simulink model "sensorFusionWithControlBackup"  (R2024a)
settings: Solver=FixedStepAuto  StartTime=0.0  StopTime=inf  FixedStep=controlRate  RelTol=1e-3  EnableMultiTasking=on
InitFcn:
  | motorParamsDD = Simulink.data.dictionary.open('motorParametersData.sldd');
  | robotParamsDD = Simulink.data.dictionary.open('robotModelData.sldd');
  | controlParamsDD = Simulink.data.dictionary.open('controlVariablesData.sldd');
  | modelParamsDD = Simulink.data.dictionary.open('modelConfigData.sldd');
  | sectMotor = getSection(motorParamsDD,'Design Data');
  | sectRobot = getSection(robotParamsDD,'Design Data');
  | sectControl = getSection(controlParamsDD,'Design Data');
  | sectModel = getSection(modelParamsDD,'Design Data');
  | 
  | %% Physical Parameters
  | M = getValue(getEntry(sectRobot,'massOfCart'));    % mass of cart
  | m = getValue(getEntry(sectRobot,'massOfPendulum'));    % mass of pendulum
  | L = getValue(getEntry(sectRobot,'lengthToPendulumCenterOfMass'));    % length to pendulum center of mass
  | g = 9.81;   % gravity
  | I = getValue(getEntry(sectRobot,'inertiaOfPendulum'));  % inertia of pendulum
  | r = getValue(getEntry(sectRobot,'wheelRadius'));   % 5 cm wheel radius
  | 
  | % Servo motor state: i, omega
  | Rm = getValue(getEntry(sectMotor,'armatureResistance')); % motor resistance
  | Lm = getValue(getEntry(sectMotor,'armatureInductance')); % motor coil inductance
  | Km = getValue(getEntry(sectMotor,'motorTorqueConstantKm')); % motor torque constant
  | Kb = getValue(getEntry(sectMotor,'backEMFConstantKb')); % motor electrical consant
  | Kf = getValue(getEntry(sectMotor,'viscousFriction')); % viscous friction
  | J = getValue(getEntry(sectMotor,'motorInertia'));  % inertia of rotor
  | 
  | 
  | Q_lqr_temp = getValue(getEntry(sectControl,'Q_lqr'));
  | R_lqr_temp = getValue(getEntry(sectControl,'R_lqr'));
  | Q_aug_lqr_temp = getValue(getEntry(sectControl,'Q_aug_lqr'));
  | R_aug_lqr_temp = getValue(getEntry(sectControl,'R_aug_lqr'));
  | 
  | % States are x, dx/dt, phi, dphi/dt
  | % Outputs are x position and tilt angle
  | 
  | % Linearized state-space model of inverted pendulum
  | I_tot = m*L^2+I;
  | p = m^2*L^2 - I_tot*(M+m);
  | A_pend = [0 1 0 0;
  |           0 0 (m^2 * g * L^2)/p 0;
  |           0 0 0 1;
  |           0 0 -(M+m)/(m*L)*m^2*L^2*g/p 0];
  | 
  | B_pend = [0; -I_tot/p; 0; 1/(m*L)*(1+(M+m)*I_tot/p)];
  | 
  | C_pend = [1 0 0 0;
  |           0 0 1 0];
  | D_pend = zeros(2,1);
  | 
  | % Discretize System - for the augmented system
  | dt = getValue(getEntry(sectModel,'stateEstRate'));
  | sysd = c2d(ss(A_pend, B_pend, C_pend, D_pend), dt);
  | Ad_pend = single(sysd.A);
  | Bd_pend = single(sysd.B);
  | Cd_pend = single(sysd.C);
  | Dd_pend = single(sysd.D);
  | 
  | % LQR Controller - for the augmented system
  | % Q_lqr = diag([1/0.02^2 1/0.1^2 1/(10*pi/180)^2 1/0.1^2]);
  | % R_lqr = 1;
  | [K_lqr, ~, ~] = dlqr(Ad_pend, Bd_pend, Q_lqr_temp, R_lqr_temp);
  | K_lqr = single(K_lqr);
  | 
  | % State-space model: output is torque = Km * i
  | A_motor = [-Rm/L,   -Kb/Lm;
  |             Km/J, -Kf/J];
  | B_motor = [1/Lm;
  |            0];
  | C_motor = [Km*(1/r), 0];  % Output is torque = Km * i
  | D_motor = 0;
  | 
  | % Augment System: Force = torque / r
  | % States are x, dx/dt, phi, dphi/dt, i, w
  | % Outputs are x position and tilt angle
  | 
  | A_aug = [A_pend, B_pend*C_motor;
  |          zeros(2,4), A_motor];
  | 
  | B_aug = [B_pend*D_motor; B_motor];
  | 
  | C_aug = [C_pend, D_pend*C_motor];
  | n_aug = size(A_aug,1);
  | 
  | 
  | % Discretize System - for the augmented system
  | sysd = c2d(ss(A_aug, B_aug, C_aug, 0), dt);
  | Ad_aug = single(sysd.A);
  | Bd_aug = single(sysd.B);
  | Cd_aug = single(sysd.C);
  | 
  | clear J Kt M m l g I r Q_lqr_temp R_lqr_temp dt
  | clear Rm Lm Km Kb Kf J
  | clear motorParamsDD robotParamsDD controlParamsDD modelParamsDD sectMotor sectRobot sectControl sectModel
  | 
  | 
  | % LQR Controller - for the augmented system
  | % Q_aug = diag([1/0.02^2 1/0.1^2 1/(10*pi/180)^2 1/0.1^2 1 1]);
  | % R_aug_lqr = 1;
  | [K_aug_lqr, ~, ~] = dlqr(Ad_aug, Bd_aug, Q_aug_lqr_temp, R_aug_lqr_temp);
  | K_aug_lqr = single(K_aug_lqr);
  | % K_aug_lqr = single([0.0 0.0 -39.4009209 -5.59002447 0.293991983 -0.0311870389])
  | 
  | clear Q_aug_lqr_temp R_aug_lqr_temp
  | 
  | % % Kalman Filter - for the augmented system
  | % Q_kf = diag([0.02 0.02 0.02 0.02]);   % Slightly higher process noise
  | % Q_kf_aug = diag([0.02 0.02 0.02 0.02 0.02 0.02]);   % Slightly higher process noise
  | % R_kf = 0.01*diag([0.001 0.001]);                 % Lower measurement noise (trust sensors more)
undefined symbols (not defined in the file): accelToUnit, angleEstRate, controlRate, CPR, D_min, DiscIntNeverNeededParam, Dmin, gyroToUnit, MaxMotorVoltage, Q_ang_kf, R_ang_kf, stateEstRate, wheelBase, wheelRadius
libraries: stm32f4xxblockslib x13, dspstat3 x6, stm32blockslib x2, stm32f7xxblockslib x2, slpidlib x1
settings Model: DataDictionary=globalData.sldd  VariantConfigurationObject=RobotVariantConfig  STM32="{\"DigitalPortWrite\":[{\"ID\":\"sensorFusionWithControlBackup:191\"},{\"ID\":\"sensorFusionWithControlBackup:197\"},{\"ID\":\"sensorFusionWithControlBackup:199\"},{\"ID\":\"sensorFusionWithControlBackup:201\"},{\"ID\":\"sensorFusionWithControlBackup:203\"},{\"ID\":\"sensorFusionWithControlBackup:667\"},{\"ID\":\"sensorFusionWithControlBackup:668\"},{\"ID\":\"sensorFusionWithControlBackup:669\"},{\"ID\":\"sensorFusionWithControlBackup:670\"},{\"ID\":\"sensorFusionWithControlBackup:778\"},{\"ID\":\"sensorFusionWithControlBackup:779\"},{\"ID\":\"sensorFusionWithControlBackup:780\"},{\"ID\":\"sensorFusionWithControlBackup:781\"}],\"PWMOutput\":[{\"ID\":\"sensorFusionWithControlBackup:205\"},{\"ID\":\"sensorFusionWithControlBackup:189\"}],\"EncoderBlock\":[{\"ID\":\"sensorFusionWithControlBackup:932\"},{\"ID\":\"sensorFusionWithControlBackup:935\"}],\"I2CControllerRead\":[{\"ID\":\"sensorFusionWithControlBackup:63:801\"},{\"ID\":\"sensorFusionWithControlBackup:63:802\"},{\"ID\":\"sensorFusionWithControlBackup:63:803\"},{\"ID\":\"sensorFusionWithControlBackup:63:804\"},{\"ID\":\"sensorFusionWithControlBackup:63:799\"},{\"ID\":\"sensorFusionWithControlBackup:63:800\"},{\"ID\":\"sensorFusionWithControlBackup:63:813\"},{\"ID\":\"sensorFusionWithControlBackup:63:814\"},{\"ID\":\"sensorFusionWithControlBackup:78:799\"},{\"ID\":\"sensorFusionWithControlBackup:78:800\"},{\"ID\":\"sensorFusionWithControlBackup:78:801\"},{\"ID\":\"sensorFusionWithControlBackup:78:802\"},{\"ID\":\"sensorFusionWithControlBackup:78:803\"},{\"ID\":\"sensorFusionWithControlBackup:78:804\"},{\"ID\":\"sensorFusionWithControlBackup:78:812\"},{\"ID\":\"sensorFusionWithControlBackup:78:813\"},{\"ID\":\"sensorFusionWithControlBackup:78:814\"}],\"I2CControllerWrite\":[{\"ID\":\"sensorFusionWithControlBackup:63:815\"},{\"ID\":\"sensorFusionWithControlBackup:63:816\"},{\"ID\":\"sensorFusionWithControlBackup:78:815\"},{\"ID\":\"sensorFusionWithControlBackup:78:816\"},{\"ID\":\"sensorFusionWithControlBackup:78:817\"}]}"  SimulationMode=external  Creator=Peter  LastModifiedBy=Peter
settings OptimizationCC: EnhancedBackFolding=on  PassReuseOutputArgsAs=Individual arguments  ZeroExternalMemoryAtStartup=off  ZeroInternalMemoryAtStartup=off  MaxStackSize=64  OptimizeBlockOrder=speed  DifferentSizesBufferReuse=on  OptimizationCustomize=off  EfficientTunableParamExpr=on
settings DebuggingCC: ParameterTunabilityLossMsg=error
settings HardwareCC: ProdBitPerPointer=32  ProdBitPerSizeT=32  ProdBitPerPtrDiffT=32  ProdLargestAtomicInteger=Long  ProdLargestAtomicFloat=Double  ProdWordSize=32  ProdLongLongMode=on  ProdHWDeviceType=ARM Compatible->ARM Cortex-M
settings SFSimCC: MATLABDynamicMemAlloc=off
settings RTWCC: Description=Embedded Coder  SystemTargetFile=ert.tlc  HardwareBoard=STM32F7xx Based (Single precision FPU)  TemplateMakefile=ert_default_tmf  Toolchain=GNU Tools for ARM Embedded Processors
settings CodeAppCC: ForceParamTrailComments=on  IgnoreCustomStorageClasses=off  OperatorAnnotations=on  SimulinkDataObjDesc=on  SFDataObjDesc=on  InsertBlockDesc=on
settings ERTTargetCC: TargetLangStandard=C99 (ISO)  CodeReplacementLibrary=ARM Cortex-M  ExtMode=on  ExtModeTransport=3  ExtModeStaticAlloc=on  ExtModeStaticAllocSize=2048  ExtModeMexFile=ext_xcp  ExtModeMexArgs=1 'COM11' 115200  ExtModeIntrfLevel=Level2 - Open

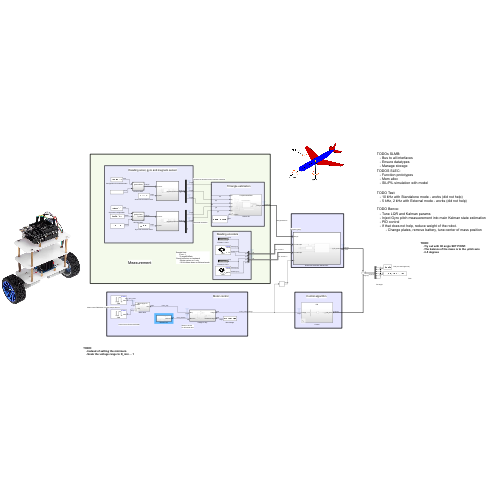
[thumbnail: Simulink's stored preview of the top-level diagram]
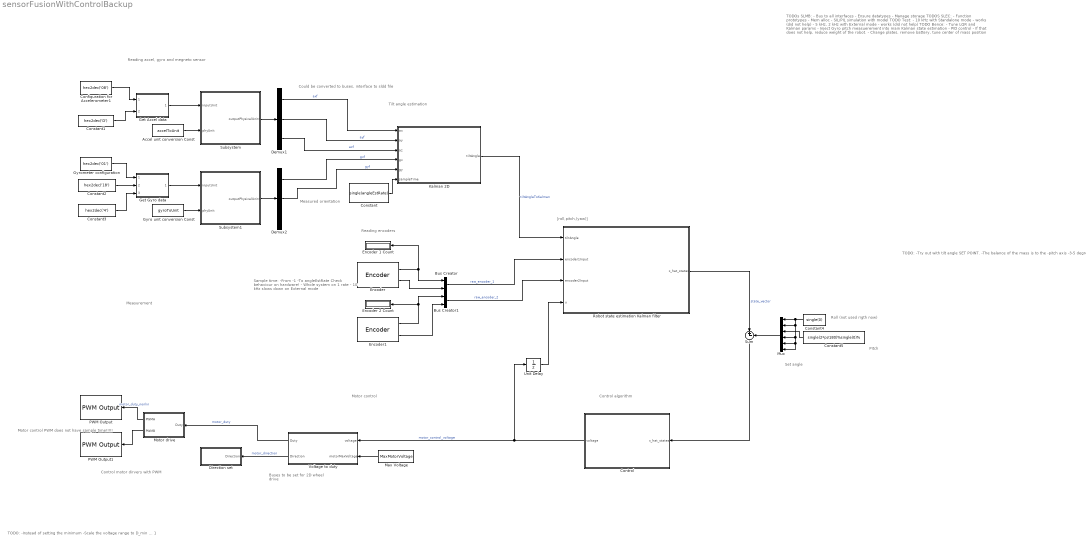
== system sensorFusionWithControlBackup ==
  note: Pitch
  note: Roll (not used rigth now)
  note: Set angle
  note: TODO:
      | -Try out with tilt angle SET POINT.
      | -The balance of the mass is to the -pitch axis
      | -3-5 degrees
  note: Measured orientation
  note: TODOs SLMB:
      | - Bus to all interfaces
      | - Ensure datatypes
      | - Manage storage
      | TODOS SLEC:
      | - Function prototypes
      | - Mem alloc
      | - SIL/PIL simulation with model
      |
      | TODO Test:
      | - 10 kHz with Standalone mode - works (did not help)
      | - 5 kHz, 2 kHz with External mode - works (did not help)
      |
      | TODO Bence:
      | - Tune LQR and Kalman params
      | - Inject Gyro pitch measuerement into main Kalman state estimation
      | - PID control
      | - If that does not help, reduce weight of the robot.
      | - Change plates, remove battery, tune center of mass position
  note: Motor control PWM does not have sample time!!!!!
  note: Sample time:
      | -From -1
      | -To angleEstRate
      | Check behaviour on hardware!
      | - Whole system on 1 rate
      | - 10 kHz slows down on External mode
  note: Measurement
  note: Motor control
  note: Tilt angle estimation
  note: Buses to be set
      | for 2D wheel drive
  note: Control motor dirvers with PWM
  note: Could be converted to buses, interface to sldd file
  note: Reading accel, gyro and megneto sensor
  note: Control algorithm
  note: TODO:
      | -Instead of setting the minimum
      | -Scale the voltage range to D_min ... 1
  note: [roll,pitch,(yaw)]
  note: Reading encoders
  Accel unit conversion Const : Constant  Value=accelToUnit  OutDataTypeStr=single
  Bus Creator : BusCreator  Inputs=2
  Bus Creator1 : BusCreator  Inputs=2
  Configuration for Accelerometer1 : Constant  Value=hex2dec('08')  OutDataTypeStr=uint8
  Constant : Constant  Value=single(angleEstRate)  OutDataTypeStr=single
  Constant1 : Constant  Value=hex2dec('D')  OutDataTypeStr=uint8
  Constant2 : Constant  Value=hex2dec('18')
  Constant3 : Constant  Value=hex2dec('4')
  Constant4 : Constant  Value=single(0)
  Constant5 : Constant  Value=single(2*pi/180)%single(0)%
  Control : Subsystem  Variant=on  VariantControl=Subsystem2  VariantActivationTime=inherit from Simulink.VariantControl
  Demux1 : Demux  Outputs=3
  Demux2 : Demux  Outputs=3
  Direction set : Subsystem  TreatAsAtomicUnit=on  SystemSampleTime=controlRate
  Encoder : stm32blockslib/Encoder  TimerModule=TIM1  EnableResetInput=off  OutputDirection=on  SampleTime=angleEstRate
      settings: LibrarySourceBlock=stm32f7xxblockslib/Encoder
  Encoder 1 Count : Display
      settings: Format=hex (Stored Integer)
  Encoder 2 Count : Display
      settings: Format=hex (Stored Integer)
  Encoder1 : stm32blockslib/Encoder  TimerModule=TIM3  EnableResetInput=off  OutputDirection=on  SampleTime=angleEstRate
      settings: LibrarySourceBlock=stm32f7xxblockslib/Encoder
  Get Accel data : Subsystem  TreatAsAtomicUnit=on  SystemSampleTime=angleEstRate  ReferencedSubsystem=getAccelData
  Get Gyro data : Subsystem  TreatAsAtomicUnit=on  SystemSampleTime=angleEstRate  ReferencedSubsystem=getGyroData
  Gyro unit conversion Const : Constant  Value=gyroToUnit  OutDataTypeStr=single
  Gyrometer configuration : Constant  Value=hex2dec('01')  OutDataTypeStr=uint8
  Kalman 2D : Subsystem  Variant=on  VariantControl=Kalman 2D  VariantActivationTime=inherit from Simulink.VariantControl
  Max Voltage : Constant  Value=MaxMotorVoltage  OutDataTypeStr=single
  Motor drive : Subsystem  Variant=on  VariantControl=Motor drive  VariantActivationTime=inherit from Simulink.VariantControl
  Mux : Mux  Inputs=6
  PWM Output : stm32f7xxblockslib/PWM Output  TimerModule=TIM8  DutycycleUnits=Percentage  EnableChannel1=off  EnableChannel2=off  EnableChannel3=on  EnableChannel4=off  EnableChannel5=off  EnableChannel6=off  EnableCounterInput=off  EnableMainOutputInput=off  EnableFrequencyInput=off  SetRCAfterCE=off  OutputDirection=off  OutputMainOutputEnableStatus=off  SampleTime=0.1  EnableSimPort=off  EnableUpdateEvent=off  EnableCaptureCompare1Event=off  EnableCaptureCompare2Event=off  EnableCaptureCompare3Event=off  EnableCaptureCompare4Event=off  EnableTriggerEvent=off  EnableBreakEvent=off  EnableBreakEvent2=off  ProcessorFamily=STM32F7  hoistedMaskSrc=ECSoC/ECSimCodegen/PWM Output
  PWM Output1 : stm32f7xxblockslib/PWM Output  TimerModule=TIM8  DutycycleUnits=Percentage  EnableChannel1=off  EnableChannel2=off  EnableChannel3=off  EnableChannel4=on  EnableChannel5=off  EnableChannel6=off  EnableCounterInput=off  EnableMainOutputInput=off  EnableFrequencyInput=off  SetRCAfterCE=off  OutputDirection=off  OutputMainOutputEnableStatus=off  SampleTime=0.1  EnableSimPort=off  EnableUpdateEvent=off  EnableCaptureCompare1Event=off  EnableCaptureCompare2Event=off  EnableCaptureCompare3Event=off  EnableCaptureCompare4Event=off  EnableTriggerEvent=off  EnableBreakEvent=off  EnableBreakEvent2=off  ProcessorFamily=STM32F7  hoistedMaskSrc=ECSoC/ECSimCodegen/PWM Output
  Robot state estimation Kalman filter : Subsystem  TreatAsAtomicUnit=on  SystemSampleTime=stateEstRate
  Subsystem : Subsystem  TreatAsAtomicUnit=on  SystemSampleTime=angleEstRate
  Subsystem1 : Subsystem  TreatAsAtomicUnit=on  SystemSampleTime=angleEstRate
  Sum : Sum  Inputs=|+-
  Unit Delay : UnitDelay  SampleTime=controlRate  HasFrameUpgradeWarning=on
  Voltage to duty : Subsystem  TreatAsAtomicUnit=on  SystemSampleTime=controlRate
  wires:
  Motor drive/1(PWMA) -> PWM Output/1  "motor_duty_nonlin"
  Motor drive/2(PWMB) -> PWM Output1/1
  Voltage to duty/1(Duty) -> Motor drive/1(Duty)  "motor_duty"
  Voltage to duty/2(Direction) -> Direction set/1(Direction)  "motor_direction"
  Max Voltage/1 -> Voltage to duty/2(motorMaxVoltage)
  Gyro unit conversion Const/1 -> Subsystem1/2(phyUnit)
  Subsystem1/1(outputPhysicalUnits) -> Demux2/1
  Gyrometer configuration/1 -> Get Gyro data/1
  Get Gyro data/1 -> Subsystem1/1(inputUnit)
  Demux1/1 -> Kalman 2D/1(ax)  "axf"
  Demux1/2 -> Kalman 2D/2(ay)  "ayf"
  Demux1/3 -> Kalman 2D/3(az)  "azf"
  Constant/1 -> Kalman 2D/6(sampleTime)
  Get Accel data/1 -> Subsystem/1(inputUnit)
  Accel unit conversion Const/1 -> Subsystem/2(phyUnit)
  Subsystem/1(outputPhysicalUnits) -> Demux1/1
  Control/1(voltage) -> Voltage to duty/1(voltage), Unit Delay/1  "motor_control_voltage"
  Demux2/1 -> Kalman 2D/4(gx)  "gxf"
  Demux2/2 -> Kalman 2D/5(gy)  "gyf"
  Constant1/1 -> Get Accel data/2
  Configuration for Accelerometer1/1 -> Get Accel data/1
  Constant2/1 -> Get Gyro data/2
  Constant3/1 -> Get Gyro data/3
  Sum/1 -> Control/1(x_hat_states)
  Mux/1 -> Sum/2
  Constant5/1 -> Mux/3
  Bus Creator/1 -> Robot state estimation Kalman filter/2(encoder1Input)  "raw_encoder_1"
  Kalman 2D/1(tiltAngle) -> Robot state estimation Kalman filter/1(tiltAngle)  "tiltAngleToKalman"
  Unit Delay/1 -> Robot state estimation Kalman filter/4(u)
  Bus Creator1/1 -> Robot state estimation Kalman filter/3(encoder2Input)  "raw_encoder_2"
  Robot state estimation Kalman filter/1(x_hat_states) -> Sum/1  "state_vector"
  Encoder/2 -> Bus Creator/2
  Encoder1/1 -> Bus Creator1/1, Encoder 2 Count/1
  Encoder1/2 -> Bus Creator1/2
  Encoder/1 -> Bus Creator/1, Encoder 1 Count/1
  Constant4/1 -> Mux/6, Mux/5, Mux/4, Mux/2, Mux/1

== system sensorFusionWithControlBackup/Control ==
  x_hat_states : Inport  OutDataTypeStr=single
  LQR : Subsystem  TreatAsAtomicUnit=on  SystemSampleTime=controlRate  VariantControl=controlAlgCtrl == 1
  LQR_with_Motor : Subsystem  TreatAsAtomicUnit=on  SystemSampleTime=controlRate  VariantControl=controlAlgCtrl == 2
  MPC : Subsystem  VariantControl=controlAlgCtrl == 3
  PID : Subsystem  VariantControl=controlAlgCtrl == 4
  voltage : Outport  OutDataTypeStr=single

== system sensorFusionWithControlBackup/Direction set ==
  note: Lower the threshold or disable this
  note: A/B inputs for direction:
      | IN1 = L, IN2 = H = CCW
      | IN1 = H, IN2 = L = CW
  Direction : Inport  OutDataTypeStr=int8
  Config for STANDBY : Constant  Value=hex2dec('01')  OutDataTypeStr=uint8
  Digital Port Write : stm32f4xxblockslib/Digital Port Write  PortName=GPIOF  PinNumber=[13]  ReadOperation=off  IOAsArray=off  EnableSimPort=off  hoistedMaskSrc=ECSoC/ECSimCodegen/Digital Port Write
      settings: LibrarySourceBlock=stm32f7xxblockslib/Digital Port Write
  If : If  ElseIfExpressions=u1 < 0, u1 == 0  ShowElse=off
  MotorForward : Subsystem  TreatAsAtomicUnit=on
  MotorReverse : Subsystem  TreatAsAtomicUnit=on
  MotorStop : Subsystem  TreatAsAtomicUnit=on
  wires:
  Config for STANDBY/1 -> Digital Port Write/1
  Direction/1 -> If/1
  If/2 -> MotorReverse/Action
  If/1 -> MotorForward/Action
  If/3 -> MotorStop/Action

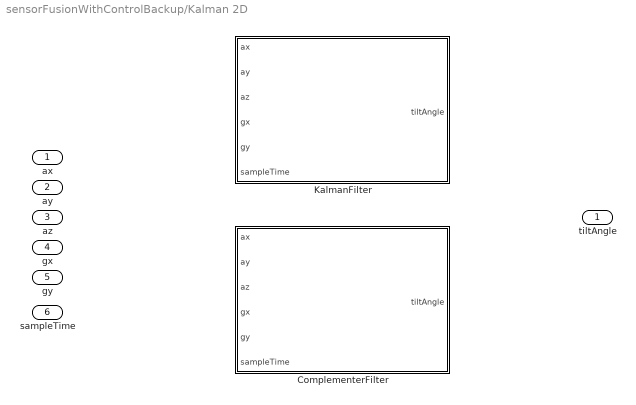
== system sensorFusionWithControlBackup/Kalman 2D ==
  ax : Inport
  ay : Inport  Port=2
  az : Inport  Port=3
  gx : Inport  Port=4
  gy : Inport  Port=5
  sampleTime : Inport  Port=6
  ComplementerFilter : Subsystem  TreatAsAtomicUnit=on  SystemSampleTime=controlRate  VariantControl=tiltEstCtrl == 2
  KalmanFilter : Subsystem  TreatAsAtomicUnit=on  SystemSampleTime=angleEstRate  VariantControl=tiltEstCtrl == 1
  tiltAngle : Outport

== system sensorFusionWithControlBackup/Motor drive ==
  Duty : Inport  OutDataTypeStr=single
  Motor drive 1D : Subsystem  TreatAsAtomicUnit=on  SystemSampleTime=controlRate  VariantControl=motorDimCtrl == 1
  Motor drive 2D : Subsystem  VariantControl=motorDimCtrl == 2
  PWMA : Outport  OutDataTypeStr=single
  PWMB : Outport  Port=2  OutDataTypeStr=single

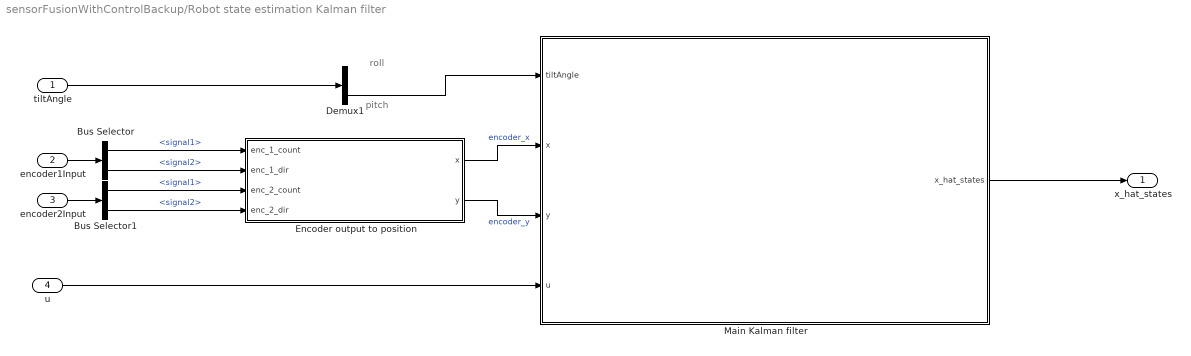
== system sensorFusionWithControlBackup/Robot state estimation Kalman filter ==
  note: pitch
  note: roll
  tiltAngle : Inport
  encoder1Input : Inport  Port=2
  encoder2Input : Inport  Port=3
  u : Inport  Port=4
  Bus Selector : BusSelector  OutputSignals=signal1,signal2
  Bus Selector1 : BusSelector  OutputSignals=signal1,signal2
  Demux1 : Demux  Outputs=2
  Encoder output to position : Subsystem  Variant=on  VariantControl=Encoder output to position  VariantActivationTime=inherit from Simulink.VariantControl
  Main Kalman filter : Subsystem  Variant=on  VariantControl=Subsystem1  VariantActivationTime=inherit from Simulink.VariantControl
  x_hat_states : Outport  OutDataTypeStr=single
  wires:
  tiltAngle/1 -> Demux1/1
  Main Kalman filter/1(x_hat_states) -> x_hat_states/1
  Bus Selector/1 -> Encoder output to position/1(enc_1_count)  "<signal1>"
  Bus Selector/2 -> Encoder output to position/2(enc_1_dir)  "<signal2>"
  Encoder output to position/1(x) -> Main Kalman filter/2(x)  "encoder_x"
  Encoder output to position/2(y) -> Main Kalman filter/3(y)  "encoder_y"
  u/1 -> Main Kalman filter/4(u)
  Demux1/2 -> Main Kalman filter/1(tiltAngle)
  encoder1Input/1 -> Bus Selector/1
  encoder2Input/1 -> Bus Selector1/1
  Bus Selector1/1 -> Encoder output to position/3(enc_2_count)  "<signal1>"
  Bus Selector1/2 -> Encoder output to position/4(enc_2_dir)  "<signal2>"

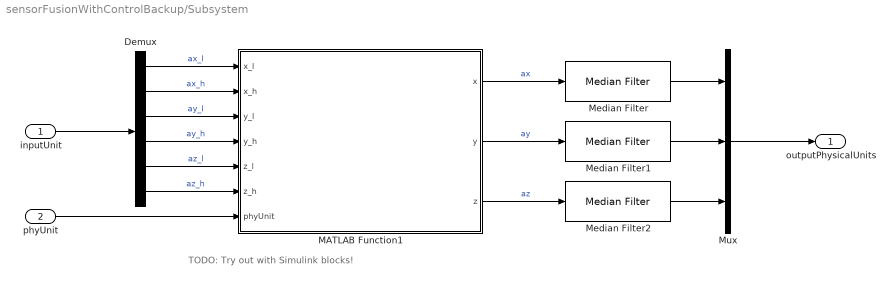
== system sensorFusionWithControlBackup/Subsystem ==
  note: TODO: Try out with Simulink blocks!
  inputUnit : Inport
  phyUnit : Inport  Port=2
  Demux : Demux  Outputs=6
  MATLAB Function1 : MATLAB Function  TreatAsAtomicUnit=on
  Median Filter : dspstat3/Median Filter  WindowLength=n_median_filt  SimulateUsing=Interpreted execution
      settings: LibrarySourceBlock=|
      | dspfdesign/Median
      | Filter
  Median Filter1 : dspstat3/Median Filter  WindowLength=n_median_filt  SimulateUsing=Interpreted execution
      settings: LibrarySourceBlock=|
      | dspfdesign/Median
      | Filter
  Median Filter2 : dspstat3/Median Filter  WindowLength=n_median_filt  SimulateUsing=Interpreted execution
      settings: LibrarySourceBlock=|
      | dspfdesign/Median
      | Filter
  Mux : Mux  Inputs=3
  outputPhysicalUnits : Outport
  wires:
  Demux/5 -> MATLAB Function1/5(z_l)  "az_l"
  Demux/6 -> MATLAB Function1/6(z_h)  "az_h"
  Demux/2 -> MATLAB Function1/2(x_h)  "ax_h"
  MATLAB Function1/3(z) -> Median Filter2/1  "az"
  Demux/3 -> MATLAB Function1/3(y_l)  "ay_l"
  Demux/1 -> MATLAB Function1/1(x_l)  "ax_l"
  Demux/4 -> MATLAB Function1/4(y_h)  "ay_h"
  phyUnit/1 -> MATLAB Function1/7(phyUnit)
  MATLAB Function1/1(x) -> Median Filter/1  "ax"
  MATLAB Function1/2(y) -> Median Filter1/1  "ay"
  inputUnit/1 -> Demux/1
  Mux/1 -> outputPhysicalUnits/1
  Median Filter/1 -> Mux/1
  Median Filter1/1 -> Mux/2
  Median Filter2/1 -> Mux/3

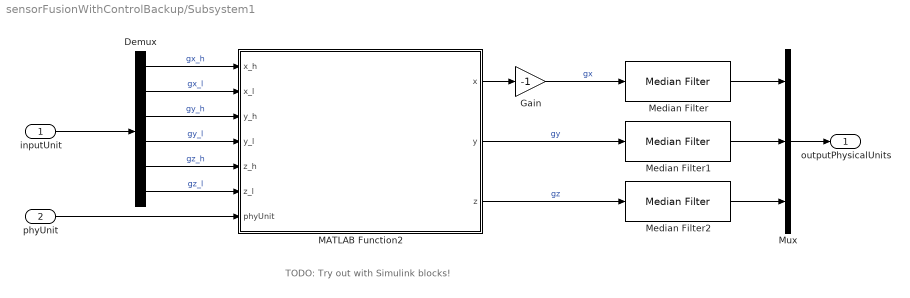
== system sensorFusionWithControlBackup/Subsystem1 ==
  note: TODO: Try out with Simulink blocks!
  inputUnit : Inport
  phyUnit : Inport  Port=2
  Demux : Demux  Outputs=6
  Gain : Gain  Gain=-1
  MATLAB Function2 : MATLAB Function  TreatAsAtomicUnit=on
  Median Filter : dspstat3/Median Filter  WindowLength=n_median_filt  SimulateUsing=Interpreted execution
      settings: LibrarySourceBlock=|
      | dspfdesign/Median
      | Filter
  Median Filter1 : dspstat3/Median Filter  WindowLength=n_median_filt  SimulateUsing=Interpreted execution
      settings: LibrarySourceBlock=|
      | dspfdesign/Median
      | Filter
  Median Filter2 : dspstat3/Median Filter  WindowLength=n_median_filt  SimulateUsing=Interpreted execution
      settings: LibrarySourceBlock=|
      | dspfdesign/Median
      | Filter
  Mux : Mux  Inputs=3
  outputPhysicalUnits : Outport
  wires:
  Mux/1 -> outputPhysicalUnits/1
  inputUnit/1 -> Demux/1
  MATLAB Function2/2(y) -> Median Filter1/1  "gy"
  MATLAB Function2/1(x) -> Gain/1
  phyUnit/1 -> MATLAB Function2/7(phyUnit)
  Demux/4 -> MATLAB Function2/4(y_l)  "gy_l"
  Demux/1 -> MATLAB Function2/1(x_h)  "gx_h"
  Demux/3 -> MATLAB Function2/3(y_h)  "gy_h"
  MATLAB Function2/3(z) -> Median Filter2/1  "gz"
  Demux/2 -> MATLAB Function2/2(x_l)  "gx_l"
  Demux/6 -> MATLAB Function2/6(z_l)  "gz_l"
  Demux/5 -> MATLAB Function2/5(z_h)  "gz_h"
  Gain/1 -> Median Filter/1  "gx"
  Median Filter/1 -> Mux/1
  Median Filter1/1 -> Mux/2
  Median Filter2/1 -> Mux/3

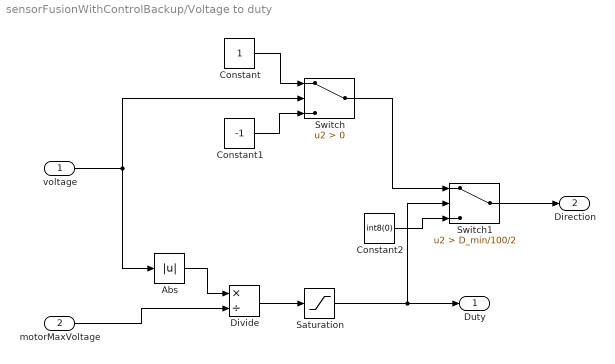
== system sensorFusionWithControlBackup/Voltage to duty ==
  voltage : Inport  OutDataTypeStr=single
  motorMaxVoltage : Inport  Port=2  OutDataTypeStr=single
  Abs : Abs  SaturateOnIntegerOverflow=off
  Constant : Constant  OutDataTypeStr=int8
  Constant1 : Constant  Value=-1  OutDataTypeStr=int8
  Constant2 : Constant  Value=int8(0)  OutDataTypeStr=int8
  Divide : Product  Inputs=*/
  Saturation : Saturate  UpperLimit=1  LowerLimit=0
  Switch : Switch  Criteria=u2 > Threshold  OutDataTypeStr=int8  SaturateOnIntegerOverflow=off  InputSameDT=off
  Switch1 : Switch  Criteria=u2 > Threshold  Threshold=D_min/100/2  OutDataTypeStr=int8  SaturateOnIntegerOverflow=off  InputSameDT=off
  Duty : Outport  OutDataTypeStr=single
  Direction : Outport  Port=2  OutDataTypeStr=int8
  wires:
  voltage/1 -> Abs/1, Switch/2
  Switch/1 -> Switch1/1
  Constant/1 -> Switch/1
  Constant1/1 -> Switch/3
  Abs/1 -> Divide/1
  motorMaxVoltage/1 -> Divide/2
  Divide/1 -> Saturation/1
  Saturation/1 -> Switch1/2, Duty/1
  Constant2/1 -> Switch1/3
  Switch1/1 -> Direction/1

== system sensorFusionWithControlBackup/Control/LQR ==
  x_hat_states : Inport
  Gain : Gain  Gain=-1
  Multiply : Gain  Gain=K_lqr  Multiplication=Matrix(K*u)
  voltage : Outport
  wires:
  x_hat_states/1 -> Multiply/1
  Multiply/1 -> Gain/1
  Gain/1 -> voltage/1

== system sensorFusionWithControlBackup/Control/LQR_with_Motor ==
  x_hat_states : Inport
  Gain : Gain  Gain=-1
  Multiply : Gain  Gain=K_aug_lqr  Multiplication=Matrix(K*u)
  voltage : Outport
  wires:
  Gain/1 -> voltage/1
  x_hat_states/1 -> Multiply/1
  Multiply/1 -> Gain/1

== system sensorFusionWithControlBackup/Control/MPC ==
  x_hat_states : Inport
  voltage : Outport

== system sensorFusionWithControlBackup/Control/PID ==
  x_hat_states : Inport
  Demux : Demux  Outputs=6
  Discrete PID Controller : slpidlib/PID Controller  Controller=PID  Form=Parallel  TimeDomain=Discrete-time  UseExternalTs=off  SampleTime=controlRate  IntegratorMethod=Forward Euler  FilterMethod=Forward Euler  ControllerParametersSource=internal  P=35  I=0.3  UseKiTs=off  D=0  UseExternalDerivativeSource=off  N=1000  UseFilter=off  TunerSelectOption=Transfer Function Based (PID Tuner App)  InitialConditionSource=internal  InitialConditionForIntegrator=0  InitialConditionForFilter=0  DifferentiatorICPrevScaledInput=0  ExternalReset=none  TrackingMode=off  Kt=1  LimitOutput=off  SatLimitsSource=internal  UpperSaturationLimit=inf  LowerSaturationLimit=-inf  LinearizeAsGain=off  AntiWindupMode=none  Kb=1  LimitIntegrator=off  UpperIntegratorSaturationLimit=inf  LowerIntegratorSaturationLimit=-inf  POutMin=[]  POutMax=[]  IOutMin=[]  IOutMax=[]  DOutMin=[]  DOutMax=[]  NOutMin=[]  NOutMax=[]  SumOutMin=[]  SumOutMax=[]  SaturationOutMin=[]  SaturationOutMax=[]  PParamMin=[]  PParamMax=[]  IParamMin=[]  IParamMax=[]  DParamMin=[]  DParamMax=[]  NParamMin=[]  NParamMax=[]  KbParamMin=[]  KbParamMax=[]  KtParamMin=[]  KtParamMax=[]  KbOutMin=[]  KbOutMax=[]  KtOutMin=[]  KtOutMax=[]  IntegratorOutMin=[]  IntegratorOutMax=[]  FilterOutMin=[]  FilterOutMax=[]  SumI1OutMin=[]  SumI1OutMax=[]  SumI2OutMin=[]  SumI2OutMax=[]  SumI3OutMin=[]  SumI3OutMax=[]  SumI4OutMin=[]  SumI4OutMax=[]  SumDOutMin=[]  SumDOutMax=[]  DifferentiatorOutMin=[]  DifferentiatorOutMax=[]  FilterDiffOutCoefMin=[]  FilterDiffOutCoefMax=[]  ReciprocalOutMin=[]  ReciprocalOutMax=[]  SumDenOutMin=[]  SumDenOutMax=[]  SumNumOutMin=[]  SumNumOutMax=[]  DivideOutMin=[]  DivideOutMax=[]  UdiffTsProdOutMin=[]  UdiffTsProdOutMax=[]  NTsProdOutMin=[]  NTsProdOutMax=[]  UintegralTsProdOutMin=[]  UintegralTsProdOutMax=[]  UngainTsProdOutMin=[]  UngainTsProdOutMax=[]  ClampingZeroOutDataTypeStr=Inherit: Inherit via back propagation  ClampingZeroOutMin=[]  ClampingZeroOutMax=[]  FilterDenConstantOutDataTypeStr=Inherit: Inherit via back propagation  FilterDenConstantOutMin=[]  FilterDenConstantOutMax=[]  PCopyOutDataTypeStr=Inherit: Inherit via back propagation  PCopyOutMin=[]  PCopyOutMax=[]  NCopyOutDataTypeStr=Inherit: Inherit via back propagation  NCopyOutMin=[]  NCopyOutMax=[]  IntegratorContinuousStateAttributes=''  IntegratorStateMustResolveToSignalObject=off  IntegratorRTWStateStorageClass=Auto  FilterContinuousStateAttributes=''  FilterStateMustResolveToSignalObject=off  FilterRTWStateStorageClass=Auto  ParallelPVariant=InternalParameters  IdealPVariant=Disabled  IVariant=InternalParameters  DVariant=InternalParameters  IntegratorVariant=Discrete  SatVariant=Disabled  AWVariant=Passthrough  PCopyVariant=Disabled  TRVariant=Disabled  FdbkBlocksVariant=Forward  IdealPFdbkVariant=Disabled  SatFdbkVariant=Disabled  DerivativeFilterVariant=Differentiator  NVariant=Passthrough  NCopyVariant=Disabled_SignalSpec  FilterICVariant=InternalICsDifferentiator  IntegratorICVariant=InternalICs  ExternalResetVariant=Disabled  TRSumVariant=Passthrough  SumFdbkVariant=Disabled  SumVariant=Sum_PID  TsampFilterVariant=InternalTs  TsampNgainVariant=Passthrough  TsampIntegralVariant=Disabled_SignalSpec  ExternalSaturationOutDataTypeStr=Inherit: Same as second input  DerivativeSourceVariant=ErrorSignal
      settings: LibrarySourceBlock=simulink/Discrete/Discrete PID Controller
  Gain : Gain
  voltage : Outport
  wires:
  x_hat_states/1 -> Demux/1
  Demux/3 -> Discrete PID Controller/1
  Discrete PID Controller/1 -> Gain/1  "pid_angle"
  Gain/1 -> voltage/1

== system sensorFusionWithControlBackup/Direction set/MotorForward ==
  note: IN1 = H, IN2 = L = CW
  Action Port : ActionPort  ActionPortLabel=if(u1 > 0)
  Config for AIN1 : Constant  Value=hex2dec('01')  OutDataTypeStr=uint8
  Config for AIN2 : Constant  Value=hex2dec('00')  OutDataTypeStr=uint8
  Config for BIN1 : Constant  Value=hex2dec('01')  OutDataTypeStr=uint8
  Config for BIN2 : Constant  Value=hex2dec('00')  OutDataTypeStr=uint8
  Digital Port Write1 : stm32f4xxblockslib/Digital Port Write  PortName=GPIOA  PinNumber=[3]  ReadOperation=off  IOAsArray=off  EnableSimPort=off  hoistedMaskSrc=ECSoC/ECSimCodegen/Digital Port Write
      settings: LibrarySourceBlock=stm32f7xxblockslib/Digital Port Write
  Digital Port Write2 : stm32f4xxblockslib/Digital Port Write  PortName=GPIOC  PinNumber=[0]  ReadOperation=off  IOAsArray=off  EnableSimPort=off  hoistedMaskSrc=ECSoC/ECSimCodegen/Digital Port Write
      settings: LibrarySourceBlock=stm32f7xxblockslib/Digital Port Write
  Digital Port Write3 : stm32f4xxblockslib/Digital Port Write  PortName=GPIOC  PinNumber=[10]  ReadOperation=off  IOAsArray=off  EnableSimPort=off  hoistedMaskSrc=ECSoC/ECSimCodegen/Digital Port Write
      settings: LibrarySourceBlock=stm32f7xxblockslib/Digital Port Write
  Digital Port Write4 : stm32f4xxblockslib/Digital Port Write  PortName=GPIOF  PinNumber=[14]  ReadOperation=off  IOAsArray=off  EnableSimPort=off  hoistedMaskSrc=ECSoC/ECSimCodegen/Digital Port Write
      settings: LibrarySourceBlock=stm32f7xxblockslib/Digital Port Write
  wires:
  Config for AIN1/1 -> Digital Port Write1/1
  Config for BIN1/1 -> Digital Port Write3/1
  Config for BIN2/1 -> Digital Port Write4/1
  Config for AIN2/1 -> Digital Port Write2/1

== system sensorFusionWithControlBackup/Direction set/MotorReverse ==
  note: IN1 = H, IN2 = L = CW
  Action Port : ActionPort  ActionPortLabel=elseif(u1 < 0)
  Config for AIN1 : Constant  Value=hex2dec('00')  OutDataTypeStr=uint8
  Config for AIN2 : Constant  Value=hex2dec('01')  OutDataTypeStr=uint8
  Config for BIN1 : Constant  Value=hex2dec('00')  OutDataTypeStr=uint8
  Config for BIN2 : Constant  Value=hex2dec('01')  OutDataTypeStr=uint8
  Digital Port Write1 : stm32f4xxblockslib/Digital Port Write  PortName=GPIOA  PinNumber=[3]  ReadOperation=off  IOAsArray=off  EnableSimPort=off  hoistedMaskSrc=ECSoC/ECSimCodegen/Digital Port Write
      settings: LibrarySourceBlock=stm32f7xxblockslib/Digital Port Write
  Digital Port Write2 : stm32f4xxblockslib/Digital Port Write  PortName=GPIOC  PinNumber=[0]  ReadOperation=off  IOAsArray=off  EnableSimPort=off  hoistedMaskSrc=ECSoC/ECSimCodegen/Digital Port Write
      settings: LibrarySourceBlock=stm32f7xxblockslib/Digital Port Write
  Digital Port Write3 : stm32f4xxblockslib/Digital Port Write  PortName=GPIOC  PinNumber=[10]  ReadOperation=off  IOAsArray=off  EnableSimPort=off  hoistedMaskSrc=ECSoC/ECSimCodegen/Digital Port Write
      settings: LibrarySourceBlock=stm32f7xxblockslib/Digital Port Write
  Digital Port Write4 : stm32f4xxblockslib/Digital Port Write  PortName=GPIOF  PinNumber=[14]  ReadOperation=off  IOAsArray=off  EnableSimPort=off  hoistedMaskSrc=ECSoC/ECSimCodegen/Digital Port Write
      settings: LibrarySourceBlock=stm32f7xxblockslib/Digital Port Write
  wires:
  Config for AIN2/1 -> Digital Port Write2/1
  Config for BIN2/1 -> Digital Port Write4/1
  Config for BIN1/1 -> Digital Port Write3/1
  Config for AIN1/1 -> Digital Port Write1/1

== system sensorFusionWithControlBackup/Direction set/MotorStop ==
  note: IN1 = H, IN2 = L = CW
  Action Port : ActionPort  ActionPortLabel=elseif( u1 == 0)
  Config for AIN1 : Constant  Value=hex2dec('00')  OutDataTypeStr=uint8
  Config for AIN2 : Constant  Value=hex2dec('00')  OutDataTypeStr=uint8
  Config for BIN1 : Constant  Value=hex2dec('00')  OutDataTypeStr=uint8
  Config for BIN2 : Constant  Value=hex2dec('00')  OutDataTypeStr=uint8
  Digital Port Write1 : stm32f4xxblockslib/Digital Port Write  PortName=GPIOA  PinNumber=[3]  ReadOperation=off  IOAsArray=off  EnableSimPort=off  hoistedMaskSrc=ECSoC/ECSimCodegen/Digital Port Write
      settings: LibrarySourceBlock=stm32f7xxblockslib/Digital Port Write
  Digital Port Write2 : stm32f4xxblockslib/Digital Port Write  PortName=GPIOC  PinNumber=[0]  ReadOperation=off  IOAsArray=off  EnableSimPort=off  hoistedMaskSrc=ECSoC/ECSimCodegen/Digital Port Write
      settings: LibrarySourceBlock=stm32f7xxblockslib/Digital Port Write
  Digital Port Write3 : stm32f4xxblockslib/Digital Port Write  PortName=GPIOC  PinNumber=[10]  ReadOperation=off  IOAsArray=off  EnableSimPort=off  hoistedMaskSrc=ECSoC/ECSimCodegen/Digital Port Write
      settings: LibrarySourceBlock=stm32f7xxblockslib/Digital Port Write
  Digital Port Write4 : stm32f4xxblockslib/Digital Port Write  PortName=GPIOF  PinNumber=[14]  ReadOperation=off  IOAsArray=off  EnableSimPort=off  hoistedMaskSrc=ECSoC/ECSimCodegen/Digital Port Write
      settings: LibrarySourceBlock=stm32f7xxblockslib/Digital Port Write
  wires:
  Config for AIN1/1 -> Digital Port Write1/1
  Config for BIN1/1 -> Digital Port Write3/1
  Config for BIN2/1 -> Digital Port Write4/1
  Config for AIN2/1 -> Digital Port Write2/1

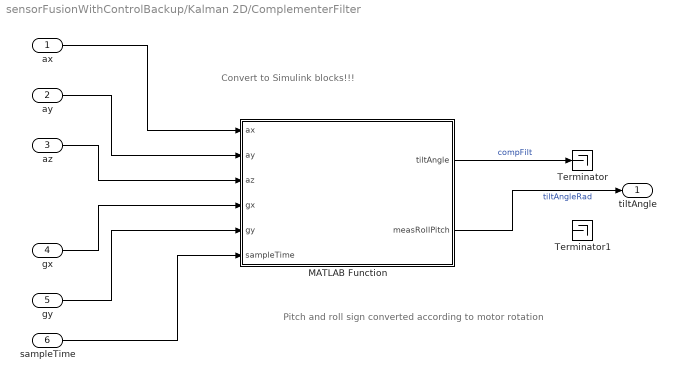
== system sensorFusionWithControlBackup/Kalman 2D/ComplementerFilter ==
  note: Convert to Simulink blocks!!!
  note: Pitch and roll sign converted according to motor rotation
  ax : Inport
  ay : Inport  Port=2
  az : Inport  Port=3
  gx : Inport  Port=4
  gy : Inport  Port=5
  sampleTime : Inport  Port=6
  MATLAB Function : MATLAB Function  TreatAsAtomicUnit=on
  Terminator : Terminator
  Terminator1 : Terminator
  tiltAngle : Outport
  wires:
  gy/1 -> MATLAB Function/5(gy)
  gx/1 -> MATLAB Function/4(gx)
  az/1 -> MATLAB Function/3(az)
  ay/1 -> MATLAB Function/2(ay)
  ax/1 -> MATLAB Function/1(ax)
  MATLAB Function/1(tiltAngle) -> Terminator/1  "compFilt"
  MATLAB Function/2(measRollPitch) -> tiltAngle/1  "tiltAngleRad"
  sampleTime/1 -> MATLAB Function/6(sampleTime)

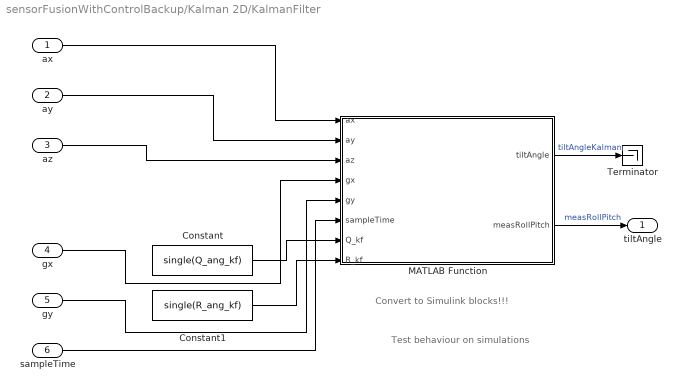
== system sensorFusionWithControlBackup/Kalman 2D/KalmanFilter ==
  note: Test behaviour on simulations
  note: Convert to Simulink blocks!!!
  ax : Inport
  ay : Inport  Port=2
  az : Inport  Port=3
  gx : Inport  Port=4
  gy : Inport  Port=5
  sampleTime : Inport  Port=6
  Constant : Constant  Value=single(Q_ang_kf)  OutDataTypeStr=single
  Constant1 : Constant  Value=single(R_ang_kf)  OutDataTypeStr=single
  MATLAB Function : MATLAB Function  TreatAsAtomicUnit=on
  Terminator : Terminator
  tiltAngle : Outport
  wires:
  ax/1 -> MATLAB Function/1(ax)
  ay/1 -> MATLAB Function/2(ay)
  az/1 -> MATLAB Function/3(az)
  gx/1 -> MATLAB Function/4(gx)
  gy/1 -> MATLAB Function/5(gy)
  MATLAB Function/1(tiltAngle) -> Terminator/1  "tiltAngleKalman"
  sampleTime/1 -> MATLAB Function/6(sampleTime)
  Constant/1 -> MATLAB Function/7(Q_kf)
  Constant1/1 -> MATLAB Function/8(R_kf)
  MATLAB Function/2(measRollPitch) -> tiltAngle/1  "measRollPitch"

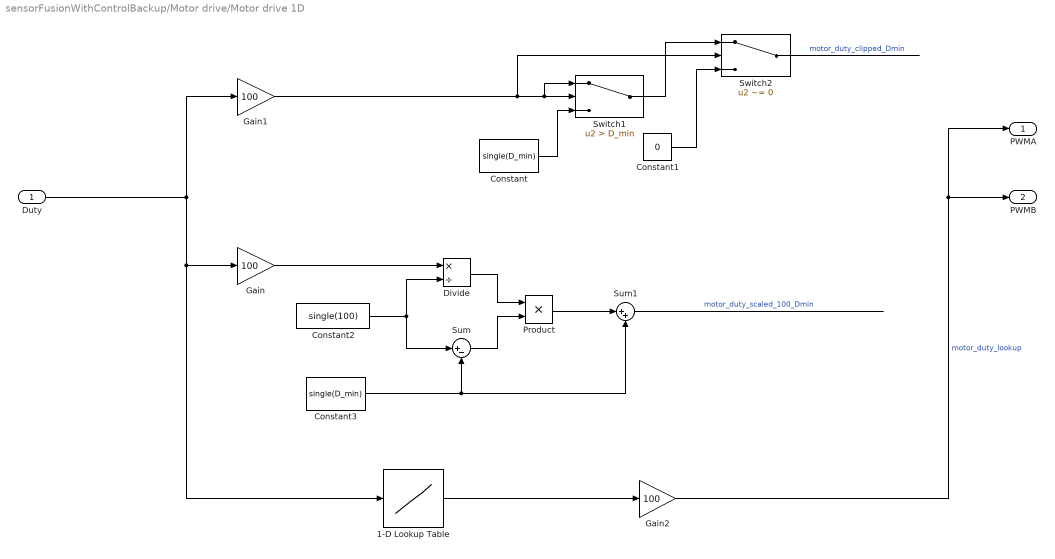
== system sensorFusionWithControlBackup/Motor drive/Motor drive 1D ==
  Duty : Inport  OutDataTypeStr=single
  1-D Lookup Table : Lookup_n-D  NumberOfTableDimensions=1  BreakpointsForDimension1=[0:0.01:1]  Table=Dmin/100*tanh([0:0.01:1]/0.05)+(100-Dmin)/100*[0:0.01:1]  InternalRulePriority=Speed  RndMeth=Simplest
  Constant : Constant  Value=single(D_min)  OutDataTypeStr=single
  Constant1 : Constant  Value=0  OutDataTypeStr=single
  Constant2 : Constant  Value=single(100)  OutDataTypeStr=single
  Constant3 : Constant  Value=single(D_min)  OutDataTypeStr=single
  Divide : Product  Inputs=*/
  Gain : Gain  Gain=100
  Gain1 : Gain  Gain=100
  Gain2 : Gain  Gain=100
  Product : Product
  Sum : Sum  Inputs=|+-
  Sum1 : Sum  Inputs=|++
  Switch1 : Switch  Criteria=u2 > Threshold  Threshold=D_min  OutDataTypeStr=single  SaturateOnIntegerOverflow=off  InputSameDT=off
  Switch2 : Switch  Criteria=u2 ~= 0  OutDataTypeStr=single  SaturateOnIntegerOverflow=off  InputSameDT=off
  PWMA : Outport  OutDataTypeStr=single
  PWMB : Outport  Port=2  OutDataTypeStr=single
  wires:
  Duty/1 -> Gain1/1, 1-D Lookup Table/1, Gain/1
  Constant/1 -> Switch1/3
  Switch1/1 -> Switch2/1
  Constant1/1 -> Switch2/3
  Constant2/1 -> Sum/1, Divide/2
  Constant3/1 -> Sum1/2, Sum/2
  Sum/1 -> Product/2
  Divide/1 -> Product/1
  Product/1 -> Sum1/1
  Sum1/1 -> ?  "motor_duty_scaled_100_Dmin"
  Switch2/1 -> ?  "motor_duty_clipped_Dmin"
  1-D Lookup Table/1 -> Gain2/1
  Gain/1 -> Divide/1
  Gain1/1 -> Switch2/2, Switch1/2, Switch1/1
  Gain2/1 -> PWMA/1, PWMB/1  "motor_duty_lookup"

== system sensorFusionWithControlBackup/Motor drive/Motor drive 2D ==
  Duty : Inport
  PWMA : Outport
  PWMB : Outport  Port=2

== system sensorFusionWithControlBackup/Robot state estimation Kalman filter/Encoder output to position ==
  enc_1_count : Inport
  enc_1_dir : Inport  Port=2
  enc_2_count : Inport  Port=3
  enc_2_dir : Inport  Port=4
  Encoder1D : Subsystem  VariantControl=encoderDimCtrl == 1
  Encoder2D : Subsystem  VariantControl=encoderDimCtrl == 2
  x : Outport  OutDataTypeStr=single
  y : Outport  Port=2  OutDataTypeStr=single

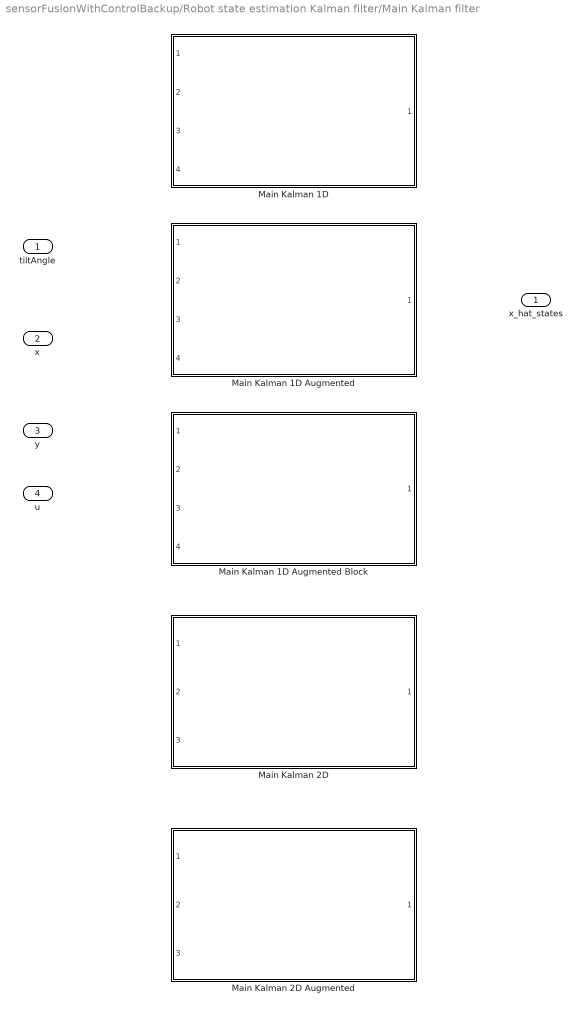
== system sensorFusionWithControlBackup/Robot state estimation Kalman filter/Main Kalman filter ==
  tiltAngle : Inport  OutDataTypeStr=single
  x : Inport  Port=2  OutDataTypeStr=single
  y : Inport  Port=3  OutDataTypeStr=single
  u : Inport  Port=4  OutDataTypeStr=single
  Main Kalman 1D : Subsystem  VariantControl=mainStateEstCtrl == 1  ReferencedSubsystem=Main_Kalman_1D
  Main Kalman 1D Augmented : Subsystem  VariantControl=mainStateEstCtrl == 2  ReferencedSubsystem=Main_Kalman_1D_Augmented
  Main Kalman 1D Augmented Block : Subsystem  VariantControl=mainStateEstCtrl == 5  ReferencedSubsystem=Main_Kalman_1D_Augmented_Block
  Main Kalman 2D : Subsystem  VariantControl=mainStateEstCtrl == 3  ReferencedSubsystem=Main_Kalman_2D
  Main Kalman 2D Augmented : Subsystem  VariantControl=mainStateEstCtrl == 4  ReferencedSubsystem=Main_Kalman_2D_Augmented
  x_hat_states : Outport  OutDataTypeStr=single

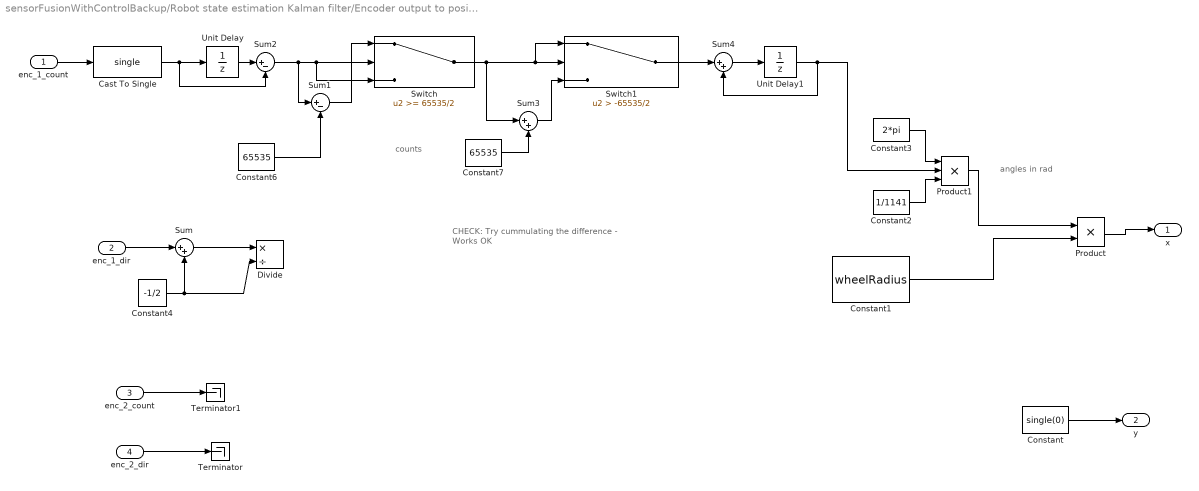
== system sensorFusionWithControlBackup/Robot state estimation Kalman filter/Encoder output to position/Encoder1D ==
  note: CHECK: Try cummulating the difference
      | 	- Works OK
  note: counts
  note: angles in rad
  enc_1_count : Inport
  enc_1_dir : Inport  Port=2
  enc_2_count : Inport  Port=3
  enc_2_dir : Inport  Port=4
  Cast To Single : DataTypeConversion  OutDataTypeStr=single  SaturateOnIntegerOverflow=off  RndMeth=Floor
  Constant : Constant  Value=single(0)  OutDataTypeStr=single
  Constant1 : Constant  Value=wheelRadius
  Constant2 : Constant  Value=1/1141  OutDataTypeStr=single
  Constant3 : Constant  Value=2*pi  OutDataTypeStr=single
  Constant4 : Constant  Value=-1/2  OutDataTypeStr=single
  Constant6 : Constant  Value=65535  OutDataTypeStr=single
  Constant7 : Constant  Value=65535  OutDataTypeStr=single
  Divide : Product  Inputs=*/  OutDataTypeStr=single
  Product : Product  OutDataTypeStr=single
  Product1 : Product  Inputs=3  OutDataTypeStr=single
  Sum : Sum  Inputs=|++  OutDataTypeStr=single
  Sum1 : Sum  Inputs=|+-
  Sum2 : Sum  Inputs=|+-  OutDataTypeStr=single  AccumDataTypeStr=single
  Sum3 : Sum  Inputs=|++
  Sum4 : Sum  Inputs=|++
  Switch : Switch  Threshold=65535/2  SaturateOnIntegerOverflow=off  InputSameDT=off
  Switch1 : Switch  Criteria=u2 > Threshold  Threshold=-65535/2  SaturateOnIntegerOverflow=off  InputSameDT=off
  Terminator : Terminator
  Terminator1 : Terminator
  Unit Delay : UnitDelay  SampleTime=-1  HasFrameUpgradeWarning=on
  Unit Delay1 : UnitDelay  SampleTime=-1  HasFrameUpgradeWarning=on
  x : Outport  OutDataTypeStr=single
  y : Outport  Port=2  OutDataTypeStr=single
  wires:
  enc_2_dir/1 -> Terminator/1
  Constant/1 -> y/1
  Product1/1 -> Product/1
  enc_2_count/1 -> Terminator1/1
  Constant2/1 -> Product1/3
  Constant3/1 -> Product1/1
  enc_1_dir/1 -> Sum/1
  Constant4/1 -> Sum/2, Divide/2
  Sum/1 -> Divide/1
  Product/1 -> x/1
  Constant6/1 -> Sum1/2
  Sum1/1 -> Switch/1
  Sum2/1 -> Sum1/1, Switch/3, Switch/2
  Unit Delay/1 -> Sum2/1
  Switch/1 -> Sum3/1, Switch1/1, Switch1/2
  Constant7/1 -> Sum3/2
  Sum3/1 -> Switch1/3
  Switch1/1 -> Sum4/1
  Sum4/1 -> Unit Delay1/1
  Unit Delay1/1 -> Sum4/2, Product1/2
  Constant1/1 -> Product/2
  Cast To Single/1 -> Sum2/2, Unit Delay/1
  enc_1_count/1 -> Cast To Single/1

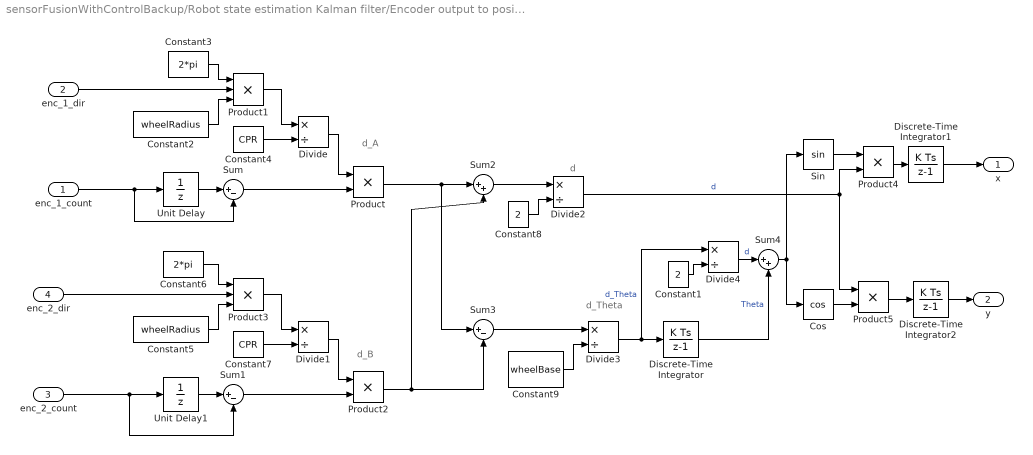
== system sensorFusionWithControlBackup/Robot state estimation Kalman filter/Encoder output to position/Encoder2D ==
  note: d_Theta
  note: d
  note: d_A
  note: d_B
  enc_1_count : Inport
  enc_1_dir : Inport  Port=2
  enc_2_count : Inport  Port=3
  enc_2_dir : Inport  Port=4
  Constant1 : Constant  Value=2
  Constant2 : Constant  Value=wheelRadius
  Constant3 : Constant  Value=2*pi
  Constant4 : Constant  Value=CPR
  Constant5 : Constant  Value=wheelRadius
  Constant6 : Constant  Value=2*pi
  Constant7 : Constant  Value=CPR
  Constant8 : Constant  Value=2
  Constant9 : Constant  Value=wheelBase
  Cos : Trigonometry  Operator=cos
  Discrete-Time Integrator : DiscreteIntegrator  SampleTime=-1  ICPrevOutput=DiscIntNeverNeededParam  ICPrevScaledInput=DiscIntNeverNeededParam
  Discrete-Time Integrator1 : DiscreteIntegrator  SampleTime=-1  ICPrevOutput=DiscIntNeverNeededParam  ICPrevScaledInput=DiscIntNeverNeededParam
  Discrete-Time Integrator2 : DiscreteIntegrator  SampleTime=-1  ICPrevOutput=DiscIntNeverNeededParam  ICPrevScaledInput=DiscIntNeverNeededParam
  Divide{,1..4} (5 alike) : Product  Inputs=*/
  Product{,2,4..5} (4 alike) : Product
  Product1 : Product  Inputs=3
  Product3 : Product  Inputs=3
  Sin : Trigonometry
  Sum : Sum  Inputs=|+-
  Sum1 : Sum  Inputs=|+-
  Sum2 : Sum  Inputs=|++
  Sum3 : Sum  Inputs=|+-
  Sum4 : Sum  Inputs=|++
  Unit Delay : UnitDelay  SampleTime=-1  HasFrameUpgradeWarning=on
  Unit Delay1 : UnitDelay  SampleTime=-1  HasFrameUpgradeWarning=on
  x : Outport  OutDataTypeStr=single
  y : Outport  Port=2  OutDataTypeStr=single
  wires:
  Discrete-Time Integrator1/1 -> x/1
  Discrete-Time Integrator2/1 -> y/1
  enc_1_count/1 -> Sum/2, Unit Delay/1
  Unit Delay/1 -> Sum/1
  Sum/1 -> Product/2
  enc_1_dir/1 -> Product1/2
  Constant2/1 -> Product1/3
  Constant3/1 -> Product1/1
  Product1/1 -> Divide/1
  Constant4/1 -> Divide/2
  Divide/1 -> Product/1
  enc_2_count/1 -> Sum1/2, Unit Delay1/1
  Sum1/1 -> Product2/2
  Constant6/1 -> Product3/1
  Constant7/1 -> Divide1/2
  Product3/1 -> Divide1/1
  Constant5/1 -> Product3/3
  Divide1/1 -> Product2/1
  enc_2_dir/1 -> Product3/2
  Unit Delay1/1 -> Sum1/1
  Product/1 -> Sum3/1, Sum2/1
  Product2/1 -> Sum3/2, Sum2/2
  Sum2/1 -> Divide2/1
  Constant8/1 -> Divide2/2
  Sum3/1 -> Divide3/1
  Constant9/1 -> Divide3/2
  Divide3/1 -> Divide4/1, Discrete-Time Integrator/1  "d_Theta"
  Discrete-Time Integrator/1 -> Sum4/2  "Theta"
  Divide2/1 -> Product4/2, Product5/1  "d"
  Constant1/1 -> Divide4/2
  Divide4/1 -> Sum4/1  "d"
  Sum4/1 -> Cos/1, Sin/1
  Sin/1 -> Product4/1
  Cos/1 -> Product5/2
  Product5/1 -> Discrete-Time Integrator2/1
  Product4/1 -> Discrete-Time Integrator1/1

== matlab function sensorFusionWithControlBackup/Subsystem/MATLAB Function1 ==
  data: x_l input uint8; x_h input uint8; x output single; y_l input uint8; y_h input uint8; z_l input uint8; z_h input uint8; y output single; z output single; phyUnit input single
function [x, y, z] = MATLAB_Function1(x_l, x_h, y_l, y_h, z_l, z_h, phyUnit)

    % Combine LSB and MSB (signed 16-bit)
    x_raw = typecast(bitor(bitshift(uint16(x_h),8), uint16(x_l)), 'int16');
    y_raw = typecast(bitor(bitshift(uint16(y_h),8), uint16(y_l)), 'int16');
    z_raw = typecast(bitor(bitshift(uint16(z_h),8), uint16(z_l)), 'int16');
    
    % Convert to physical units
    % ADXL345: 4mg/LSB (±2g range)
    x = single(x_raw) * phyUnit;
    y = single(y_raw) * phyUnit;
    z = single(z_raw) * phyUnit;
    
end

== matlab function sensorFusionWithControlBackup/Kalman 2D/ComplementerFilter/MATLAB Function ==
  data: ax input single; tiltAngle output single; ay input single; az input single; gx input single; gy input single; sampleTime input single; measRollPitch output single
function [tiltAngle, measRollPitch] = compTiltFilter(ax, ay, az, gx, gy, sampleTime)
%#codegen


dt = single(sampleTime); % Sample time
deg2rad = single(pi / 180);

% Lowpass cutoff frequency
fc = 30;

% alpha (gyro high-pass / accel low-pass) using time constant tau = 1/(2*pi*fc)
tau = 1 / (2*pi*fc);
alpha = tau / (tau + dt);   % typical complement: angle = alpha*(angle+gyro*dt) + (1-alpha)*accAngle

% Estimate roll and pitch from accelerometer
roll_meas  = -atan2(ax,az);
pitch_meas = -atan2(ay,az);
z = [roll_meas; pitch_meas];

measRollPitch = z;

% persistent state
persistent x_est initialized
if isempty(initialized)
    x_est = single([measRollPitch(1); measRollPitch(2)]); % initialize to angels from accel
    initialized = true;
end

% convert gyro to rad/s
gx_rad = gx * deg2rad; % Pitch
gy_rad = gy * deg2rad; % Roll

% integrate gyro (has offset)
x_pred = x_est + dt * [gy_rad; gx_rad];

% complementary update
x_est = alpha * x_pred + (1 - alpha) * [measRollPitch(1); measRollPitch(2)];

tiltAngle = x_est;           % [roll; pitch] in radians
end

== matlab function sensorFusionWithControlBackup/Kalman 2D/KalmanFilter/MATLAB Function ==
  data: ax input single; tiltAngle output single; ay input single; az input single; gx input single; gy input single; sampleTime input single; Q_kf input single; R_kf input single; measRollPitch output single
function [tiltAngle,measRollPitch] = kalman2D(ax, ay, az, gx, gy,sampleTime,Q_kf,R_kf)
%#codegen

persistent x P instance

dt = single(sampleTime); % Sample time
deg2rad = single(pi / 180);

% Initialize persistent state vector and covariance matrix
if isempty(instance)
    % State: [theta_x; theta_y; omega_x; omega_y]
    x = single(zeros(4, 1));
    P = single(eye(4) * 0.1);
    instance = true;
end

% System dynamics matrix
A = single([1 0 dt 0;
             0 1 0 dt;
             0 0 1  0;
             0 0 0  1]);

% Process noise covariance (tune as needed)
Q = single(Q_kf);

% Measurement matrix: we only measure [theta_x, theta_y]
H = single([1 0 0 0;
            0 1 0 0]);

% Measurement noise covariance
R = single(R_kf);

% ====== PREDICT STEP ======

% Inject new gyro measurements into angular rate state (rad/s)!!!!!!!!!!!!
x(3) = gy * deg2rad;
x(4) = gx * deg2rad;

% Can be:
   % B = single([0 0;
   %              0 0;
   %              1 0;
   %              0 1]);
   % 
   %  % ===== PREDICT STEP =====
   %  % Gyro control input (rad/s)
   %  u = [gx; gy] * deg2rad;
   % 
   %  % Predict next state
   %  x = A * x + B * u;

% Predict state and covariance
x = A * x;
P = A * P * A' + Q;

% ====== MEASUREMENT FROM ACCELEROMETER ======

% Estimate roll and pitch from accelerometer
roll_meas  = atan2(ax,az);
% pitch_meas = atan(-ax / sqrt(ay^2 + az^2));
pitch_meas = atan2(ay,az);
z = [roll_meas; pitch_meas];

measRollPitch = z;


% ====== UPDATE STEP ======
K = P * H' / (H * P * H' + R);
x = x + K * (z - H * x);
P = (eye(4) - K * H) * P;

% Output estimated [roll; pitch]
tiltAngle = x(1:2);
end

== matlab function sensorFusionWithControlBackup/Subsystem1/MATLAB Function2 ==
  data: x output single; x_h input uint8; x_l input uint8; y_h input uint8; y_l input uint8; z_h input uint8; z_l input uint8; y output single; z output single; phyUnit input single
function [x, y, z] = convert_raw_units(x_h, x_l, y_h, y_l, z_h, z_l, phyUnit)

    % Combine LSB and MSB (signed 16-bit)
    x_raw = typecast(bitor(bitshift(uint16(x_h),8), uint16(x_l)), 'int16');
    y_raw = typecast(bitor(bitshift(uint16(y_h),8), uint16(y_l)), 'int16');
    z_raw = typecast(bitor(bitshift(uint16(z_h),8), uint16(z_l)), 'int16');
    
    % Convert to physical units
    % ITG3200: 14.375 LSBs per °/sec
    x = single(x_raw) / phyUnit;
    y = single(y_raw) / phyUnit;
    z = single(z_raw) / phyUnit;
    
end
